simulink model "sim8transmitancja"  (R2013a)
settings: Solver=ode45  StartTime=0.0  StopTime=10.0  RelTol=1e-3
values from neighbouring files (symbols this model uses):
  A1 = 2    [cwiczenie8.m]    (also in cwiczenie8transmitancja.m; dawid.m)
  a1 = 4    [cwiczenie8.m]    (also in cwiczenie8transmitancja.m)
  a2 = 5    [cwiczenie8.m]    (also in cwiczenie8transmitancja.m)
  A2 = 4    [cwiczenie8.m]    (also in cwiczenie8transmitancja.m; dawid.m)
  du = 0.1*u0max    (= 0.3)    [cwiczenie8.m]    (also in cwiczenie8transmitancja.m; dawid.m)
  h10 = u0/a1    [cwiczenie8.m]    (also in cwiczenie8transmitancja.m; dawid.m = u0*u0 / (Awy*Awy*2*g))
  h20 = u0/a2    [cwiczenie8.m]    (also in cwiczenie8transmitancja.m; dawid.m = u0*u0 / (Awe*Awe*2*g))
  u0 = tabu0(i)    [cwiczenie8.m]    (also in cwiczenie8transmitancja.m; dawid.m)
settings Model: Creator=LAB320-1552  LastModifiedBy=LAB320-1552

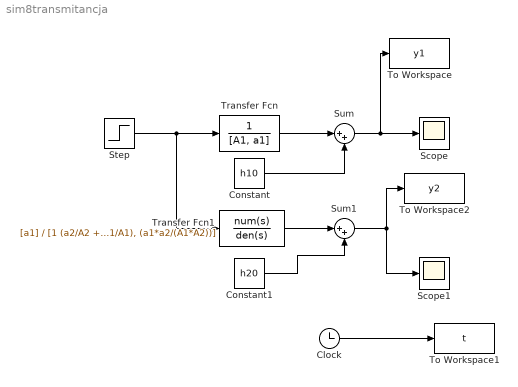
== system sim8transmitancja ==
  Clock : Clock
  Constant : Constant  Value=h10
  Constant1 : Constant  Value=h20
  Scope : Scope
  Scope1 : Scope
  Step : Step  Before=u0  After=u0+du  SampleTime=0
  Sum : Sum  Inputs=|++
  Sum1 : Sum  Inputs=|++
  To Workspace : ToWorkspace  VariableName=y1  SampleTime=-1
  To Workspace1 : ToWorkspace  VariableName=t  SampleTime=-1
  To Workspace2 : ToWorkspace  VariableName=y2  SampleTime=-1
  Transfer Fcn : TransferFcn  Denominator=[A1, a1]
  Transfer Fcn1 : TransferFcn  Numerator=[a1]  Denominator=[1 (a2/A2 + a1/A1), (a1*a2/(A1*A2))]
  wires:
  Sum/1 -> To Workspace/1, Scope/1
  Transfer Fcn/1 -> Sum/1
  Step/1 -> Transfer Fcn1/1, Transfer Fcn/1
  Constant/1 -> Sum/2
  Clock/1 -> To Workspace1/1
  Transfer Fcn1/1 -> Sum1/1
  Constant1/1 -> Sum1/2
  Sum1/1 -> To Workspace2/1, Scope1/1
